simulink model "intent_estimator_base"  (R2024b)
settings: Solver=VariableStepAuto  StartTime=0.0  StopTime=10.0  RelTol=1e-3
undefined symbols (not defined in the file): LQR
libraries: simulink_extras x1
settings Model: Creator=lukec  LastModifiedBy=lukec
settings OptimizationCC: DefaultParameterBehavior=Inlined  EnhancedBackFolding=on  PassReuseOutputArgsAs=Individual arguments  ZeroExternalMemoryAtStartup=off  ZeroInternalMemoryAtStartup=off  OptimizeBlockOrder=speed  DifferentSizesBufferReuse=on  OptimizationCustomize=off  EfficientTunableParamExpr=on
settings DebuggingCC: ParameterTunabilityLossMsg=error
settings HardwareCC: ProdBitPerPointer=32  ProdBitPerSizeT=32  ProdBitPerPtrDiffT=32  ProdLargestAtomicInteger=Long  ProdLargestAtomicFloat=Double  ProdWordSize=32  ProdHWDeviceType=ARM Compatible->ARM Cortex-M
settings SFSimCC: MATLABDynamicMemAlloc=off
settings RTWCC: Description=Embedded Coder  SystemTargetFile=ert.tlc  GenCodeOnly=on  PackageGeneratedCodeAndArtifacts=on  TemplateMakefile=ert_default_tmf  Toolchain=CMake  TargetLang=C++  HalideCodeGeneration=on
settings CodeAppCC: ForceParamTrailComments=on  IgnoreCustomStorageClasses=off  MaxIdLength=255  OperatorAnnotations=on  SimulinkDataObjDesc=on  SFDataObjDesc=on  InsertBlockDesc=on
settings ERTTargetCC: TargetLangStandard=C++17 (ISO)  CodeInterfacePackaging=C++ class  RootIOFormat=Structure reference  ERTCustomFileTemplate=example_file_process.tlc  ArrayContainerType=std::array

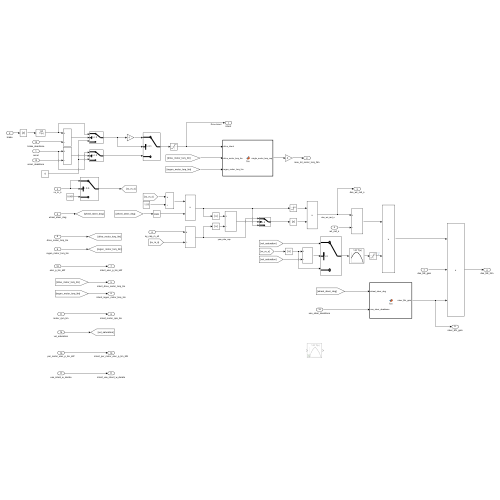
[thumbnail: Simulink's stored preview of the top-level diagram]
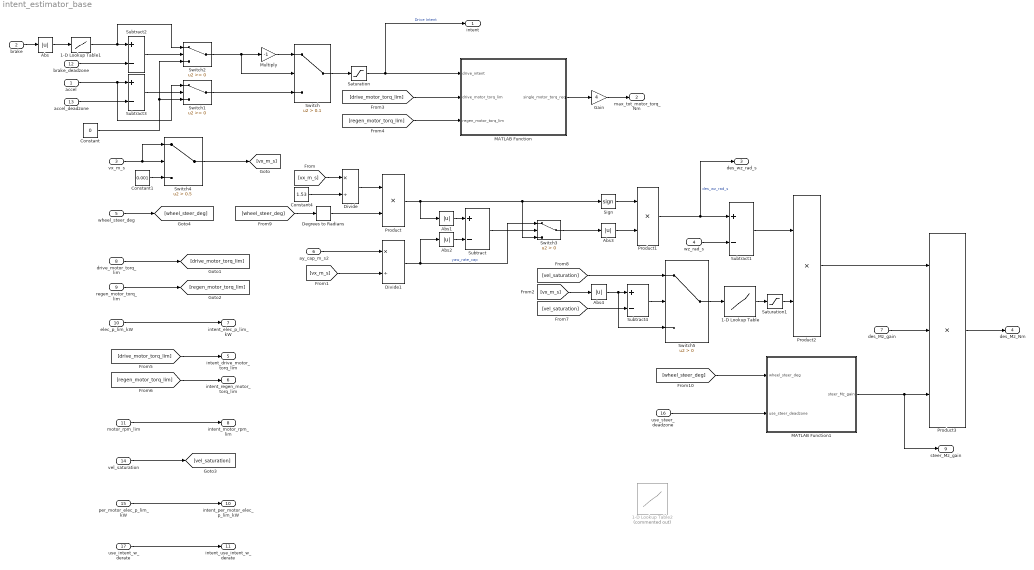
== system intent_estimator_base ==
  accel : Inport
  brake : Inport  Port=2
  vx_m_s : Inport  Port=3
  wz_rad_s : Inport  Port=4
  wheel_steer_deg : Inport  Port=5
  ay_cap_m_s2 : Inport  Port=6
  des_Mz_gain : Inport  Port=7
  drive_motor_torq_lim : Inport  Port=8
  regen_motor_torq_lim : Inport  Port=9
  elec_p_lim_kW : Inport  Port=10
  motor_rpm_lim : Inport  Port=11
  brake_deadzone : Inport  Port=12
  accel_deadzone : Inport  Port=13
  vel_saturation : Inport  Port=14
  per_motor_elec_p_lim_kW : Inport  Port=15
  use_steer_deadzone : Inport  Port=16  OutDataTypeStr=boolean
  use_intent_w_derate : Inport  Port=17  OutDataTypeStr=boolean
  1-D Lookup Table : Lookup_n-D  NumberOfTableDimensions=1  BreakpointsForDimension1="[2\t2.28282828282828\t2.56565656565657\t2.84848484848485\t3.13131313131313\t3.41414141414141\t3.69696969696970\t3.97979797979798\t4.26262626262626\t4.54545454545455\t4.82828282828283\t5.11111111111111\t5.39393939393939\t5.67676767676768\t5.95959595959596\t6.24242424242424\t6.52525252525253\t6.80808080808081\t7.09090909090909\t7.37373737373737\t7.65656565656566\t7.93939393939394\t8.22222222222222\t8.50505050505051\t8.78787878787879\t9.07070707070707\t9.35353535353535\t9.63636363636364\t9.91919191919192\t10.2020202020202\t10.4848484848485\t10.7676767676768\t11.0505050505051\t11.3333333333333\t11.6161616161616\t11.8989898989899\t12.1818181818182\t12.4646464646465\t12.7474747474747\t13.0303030303030\t13.3131313131313\t13.5959595959596\t13.8787878787879\t14.1616161616162\t14.4444444444444\t14.7272727272727\t15.0101010101010\t15.2929292929293\t15.5757575757576\t15.8585858585859\t16.1414141414141\t16.4242424242424\t16.7070707070707\t16.9898989898990\t17.2727272727273\t17.5555555555556\t17.8383838383838\t18.1212121212121\t18.4040404040404\t18.6868686868687\t18.9696969696970\t19.2525252525253\t19.5353535353535\t19.8181818181818\t20.1010101010101\t20.3838383838384\t20.6666666666667\t20.9494949494949\t21.2323232323232\t21.5151515151515\t21.7979797979798\t22.0808080808081\t22.3636363636364\t22.6464646464646\t22.9292929292929\t23.2121212121212\t23.4949494949495\t23.7777777777778\t24.0606060606061\t24.3434343434343\t24.6262626262626\t24.9090909090909\t25.1919191919192\t25.4747474747475\t25.7575757575758\t26.0404040404040\t26.3232323232323\t26.6060606060606\t26.8888888888889\t27.1717171717172\t27.4545454545455\t27.7373737373737\t28.0202020202020\t28.3030303030303\t28.5858585858586\t28.8686868686869\t29.1515151515152\t29.4343434343434\t29.7171717171717\t30]"  Table=|  ExtrapMethod=Clip  UseLastTableValue=on  InternalRulePriority=Speed  RndMeth=Simplest
      | [-143.901090552424
      | -52.1637429093211
      | 37.3991892874492
      | 124.787706037886
      | 210.001807341991
      | 293.041493199762
      | 373.906763611200
      | 452.597618576305
      | 529.114058095078
      | 603.456082167517
      | 675.623690793623
      | 745.616883973396
      | 813.435661706837
      | 879.080023993944
      | 942.549970834719
      | 1003.84550222916
      | 1062.96661817727
      | 1119.91331867904
      | 1174.68560373449
      | 1227.28347334360
      | 1277.70692750637
      | 1325.95596622282
      | 1372.03058949293
      | 1415.93079731670
      | 1457.65658969415
      | 1497.20796662526
      | 1534.58492811004
      | 1569.78747414848
      | 1602.81560474060
      | 1633.66931988638
      | 1662.34861958582
      | 1688.85350383894
      | 1713.18397264572
      | 1735.34002600616
      | 1755.32166392028
      | 1773.12888638806
      | 1788.76169340951
      | 1802.22008498462
      | 1813.50406111341
      | 1822.61362179586
      | 1829.54876703197
      | 1834.30949682176
      | 1836.89581116521
      | 1837.30771006232
      | 1835.54519351311
      | 1831.60826151756
      | 1825.49691407568
      | 1817.21115118747
      | 1806.75097285292
      | 1794.11637907204
      | 1779.30736984483
      | 1762.32394517128
      | 1743.16610505140
      | 1721.83384948519
      | 1698.32717847264
      | 1672.64609201376
      | 1644.79059010855
      | 1614.76067275701
      | 1582.55633995913
      | 1548.17759171492
      | 1511.62442802438
      | 1472.89684888750
      | 1431.99485430429
      | 1388.91844427475
      | 1343.66761879888
      | 1296.24237787667
      | 1246.64272150813
      | 1194.86864969325
      | 1140.92016243205
      | 1084.79725972451
      | 1026.49994157063
      | 966.028207970428
      | 903.382058923889
      | 838.561494431017
      | 771.566514491812
      | 702.397119106275
      | 631.053308274403
      | 557.535081996199
      | 481.842440271662
      | 403.975383100793
      | 323.933910483590
      | 241.718022420054
      | 157.327718910185
      | 70.7629999539835
      | -17.9761344485514
      | -108.889684297419
      | -201.977649592619
      | -297.240030334154
      | -394.676826522021
      | -494.288038156221
      | -596.073665236752
      | -700.033707763618
      | -806.168165736817
      | -914.477039156349
      | -1024.96032802221
      | -1137.61803233441
      | -1252.45015209294
      | -1369.45668729781
      | -1488.63763794900
      | -1609.99300404653]
  1-D Lookup Table1 : Lookup_n-D  NumberOfTableDimensions=1  BreakpointsForDimension1=[0 0.6]  Table=[0 1]  ExtrapMethod=Clip  InternalRulePriority=Speed  RndMeth=Simplest
  1-D Lookup Table2 : Lookup_n-D  Commented=on  NumberOfTableDimensions=1  BreakpointsForDimension1=LQR.V_vec(1, :)  Table=[LQR.K(1:4, 2); flip(LQR.K(1:3, 2))]'  ExtrapMethod=Clip  UseLastTableValue=on  InternalRulePriority=Speed  RndMeth=Simplest
  Abs{,1..4} (5 alike) : Abs  SaturateOnIntegerOverflow=off
  Constant : Constant  Value=0
  Constant1 : Constant  Value=0.001
  Constant4 : Constant  Value=1.53
  Degrees to Radians : simulink_extras/Transformations/Degrees to Radians
  Divide : Product  Inputs=*/
  Divide1 : Product  Inputs=*/
  Gain : Gain  Gain=4
  MATLAB Function : MATLAB Function  TreatAsAtomicUnit=on
  MATLAB Function1 : MATLAB Function  TreatAsAtomicUnit=on
  Multiply : Gain  Gain=-1
  Product : Product
  Product1 : Product
  Product2 : Product
  Product3 : Product  Inputs=3
  Saturation : Saturate  UpperLimit=1  LowerLimit=-1
  Saturation1 : Saturate  UpperLimit=2000  LowerLimit=100
  Sign : Signum
  Subtract{,1..4} (5 alike) : Sum  Inputs=+-
  Switch : Switch  Criteria=u2 > Threshold  Threshold=0.1  SaturateOnIntegerOverflow=off  InputSameDT=off
  Switch1 : Switch  SaturateOnIntegerOverflow=off  InputSameDT=off
  Switch2 : Switch  SaturateOnIntegerOverflow=off  InputSameDT=off
  Switch3 : Switch  Criteria=u2 > Threshold  SaturateOnIntegerOverflow=off  InputSameDT=off
  Switch4 : Switch  Criteria=u2 > Threshold  Threshold=0.5  SaturateOnIntegerOverflow=off  InputSameDT=off
  Switch5 : Switch  Criteria=u2 > Threshold  SaturateOnIntegerOverflow=off  InputSameDT=off
  intent : Outport
  max_tot_motor_torq_Nm : Outport  Port=2
  des_wz_rad_s : Outport  Port=3
  des_Mz_Nm : Outport  Port=4
  intent_drive_motor_torq_lim : Outport  Port=5
  intent_regen_motor_torq_lim : Outport  Port=6
  intent_elec_p_lim_kW : Outport  Port=7
  intent_motor_rpm_lim : Outport  Port=8
  steer_Mz_gain : Outport  Port=9
  intent_per_motor_elec_p_lim_kW : Outport  Port=10
  intent_use_intent_w_derate : Outport  Port=11
  wires:
  Gain/1 -> max_tot_motor_torq_Nm/1
  Switch2/1 -> Switch/2, Multiply/1
  brake/1 -> Abs/1
  Constant/1 -> Switch1/3, Switch2/3
  Switch/1 -> Saturation/1
  Saturation/1 -> intent/1, MATLAB Function/1(drive_intent)  "Drive Intent"
  Multiply/1 -> Switch/1
  MATLAB Function/1(single_motor_torq_req) -> Gain/1
  Switch1/1 -> Switch/3
  Constant4/1 -> Divide/2
  Product1/1 -> des_wz_rad_s/1, Subtract1/1  "des_wz_rad_s"
  [vx_m_s] -> Divide1/2
  Degrees to Radians/1 -> Product/2
  Divide/1 -> Product/1
  Product/1 -> Abs1/1, Switch3/3, Sign/1
  Divide1/1 -> Switch3/1, Abs2/1  "yaw_rate_cap"
  1-D Lookup Table/1 -> Saturation1/1
  Constant1/1 -> Switch4/3
  wz_rad_s/1 -> Subtract1/2
  ay_cap_m_s2/1 -> Divide1/1
  des_Mz_gain/1 -> Product3/2
  vx_m_s/1 -> Switch4/1, Switch4/2
  Switch3/1 -> Abs3/1
  Switch4/1 -> [vx_m_s]
  Subtract/1 -> Switch3/2
  Sign/1 -> Product1/1
  Abs2/1 -> Subtract/2
  Product3/1 -> des_Mz_Nm/1
  Subtract1/1 -> Product2/1
  [vx_m_s] -> Divide/1
  Abs3/1 -> Product1/2
  Abs1/1 -> Subtract/1
  Product2/1 -> Product3/1
  drive_motor_torq_lim/1 -> [drive_motor_torq_lim]
  regen_motor_torq_lim/1 -> [regen_motor_torq_lim]
  [drive_motor_torq_lim] -> MATLAB Function/2(drive_motor_torq_lim)
  [regen_motor_torq_lim] -> MATLAB Function/3(regen_motor_torq_lim)
  [drive_motor_torq_lim] -> intent_drive_motor_torq_lim/1
  [regen_motor_torq_lim] -> intent_regen_motor_torq_lim/1
  elec_p_lim_kW/1 -> intent_elec_p_lim_kW/1
  motor_rpm_lim/1 -> intent_motor_rpm_lim/1
  Abs/1 -> 1-D Lookup Table1/1
  brake_deadzone/1 -> Subtract2/2
  Subtract2/1 -> Switch2/2
  accel/1 -> Switch1/1, Subtract3/1
  Subtract3/1 -> Switch1/2
  accel_deadzone/1 -> Subtract3/2
  [vx_m_s] -> Abs4/1
  Abs4/1 -> Switch5/3, Subtract4/1
  Subtract4/1 -> Switch5/2
  vel_saturation/1 -> [vel_saturation]
  [vel_saturation] -> Subtract4/2
  [vel_saturation] -> Switch5/1
  Saturation1/1 -> Product2/2
  wheel_steer_deg/1 -> [wheel_steer_deg]
  [wheel_steer_deg] -> Degrees to Radians/1
  [wheel_steer_deg] -> MATLAB Function1/1(wheel_steer_deg)
  per_motor_elec_p_lim_kW/1 -> intent_per_motor_elec_p_lim_kW/1
  MATLAB Function1/1(steer_Mz_gain) -> steer_Mz_gain/1, Product3/3
  Switch5/1 -> 1-D Lookup Table/1
  use_steer_deadzone/1 -> MATLAB Function1/2(use_steer_deadzone)
  use_intent_w_derate/1 -> intent_use_intent_w_derate/1
  1-D Lookup Table1/1 -> Switch2/1, Subtract2/1

== matlab function intent_estimator_base/MATLAB Function ==
  data: drive_intent input; single_motor_torq_req output; drive_motor_torq_lim input; regen_motor_torq_lim input
function single_motor_torq_req = fcn(drive_intent, drive_motor_torq_lim, regen_motor_torq_lim)

    if drive_intent == 0
        single_motor_torq_req = 0;
    elseif drive_intent < 0
        single_motor_torq_req = interp1([-1 0], [regen_motor_torq_lim, 0], drive_intent);
    else
        single_motor_torq_req = interp1([0 1], [0, drive_motor_torq_lim], drive_intent);
    end

== matlab function intent_estimator_base/MATLAB Function1 ==
  data: wheel_steer_deg input; steer_Mz_gain output; use_steer_deadzone input
function steer_Mz_gain = fcn(wheel_steer_deg, use_steer_deadzone)

if use_steer_deadzone

    no_gain_deg = 2;
    full_gain_deg = 4;

    if abs(wheel_steer_deg) >= full_gain_deg
        steer_Mz_gain = 1;
    elseif abs(wheel_steer_deg) >= 0 && abs(wheel_steer_deg) <= no_gain_deg
        steer_Mz_gain = 0.01;
    else
        steer_Mz_gain = interp1([no_gain_deg full_gain_deg], [0.01 1], abs(wheel_steer_deg));
    end
    
else
    steer_Mz_gain = 1;
end
